simulink model "test_simu2"  (R2019a)
settings: Solver=VariableStepAuto  StartTime=0.0  StopTime=10.0  RelTol=1e-3
values from neighbouring files (symbols this model uses):
  b = 3.0 *10^-5    (= 3e-05)    [constants_drone.m]    (also in drone.m)
  d = 1.1*10^-6    (= 1.1e-06)    [constants_drone.m]    (also in drone.m)
  omega1 = 475    [constants_drone.m]
  omega2 = 500    [constants_drone.m]
  omega3 = 475    [constants_drone.m]
  omega4 = 475    [constants_drone.m]
undefined symbols (not defined in the file or in its folder): magnitude
settings Model: Creator=Emil  LastModifiedBy=Emil

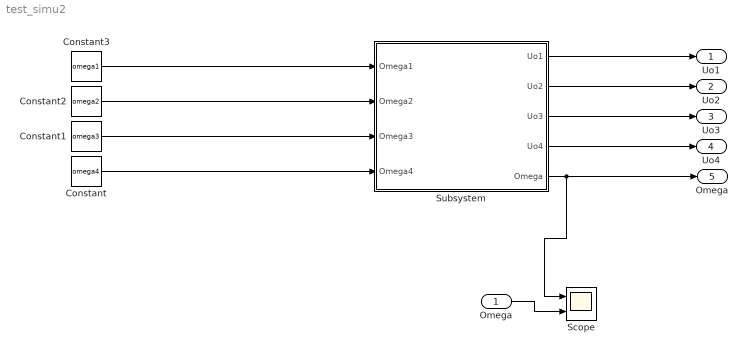
== system test_simu2 ==
  "Omega " : Inport
  Constant : Constant  Value=omega4
  Constant1 : Constant  Value=omega3
  Constant2 : Constant  Value=omega2
  Constant3 : Constant  Value=omega1
  Scope : Scope  NumInputPorts=2
  Subsystem : Subsystem
  Uo1 : Outport
  Uo2 : Outport  Port=2
  Uo3 : Outport  Port=3
  Uo4 : Outport  Port=4
  Omega : Outport  Port=5
  wires:
  Constant3/1 -> Subsystem/1(Omega1)
  Constant2/1 -> Subsystem/2(Omega2)
  Constant1/1 -> Subsystem/3(Omega3)
  Constant/1 -> Subsystem/4(Omega4)
  Subsystem/1(Uo1) -> Uo1/1
  Subsystem/2(Uo2) -> Uo2/1
  Subsystem/3(Uo3) -> Uo3/1
  Subsystem/4(Uo4) -> Uo4/1
  Subsystem/5(Omega) -> Scope/1, Omega/1
  "Omega "/1 -> Scope/2

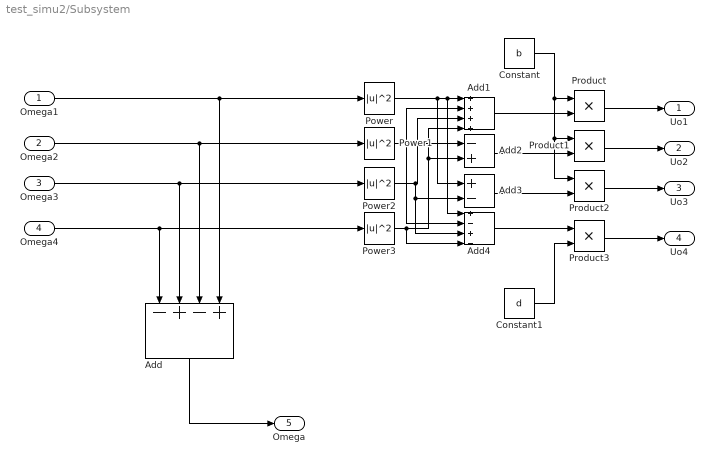
== system test_simu2/Subsystem ==
  Omega1 : Inport
  Omega2 : Inport  Port=2
  Omega3 : Inport  Port=3
  Omega4 : Inport  Port=4
  Add : Sum  Inputs=-+-+
  Add1 : Sum  Inputs=++++
  Add2 : Sum  Inputs=-+
  Add3 : Sum  Inputs=+-
  Add4 : Sum  Inputs=+-+-
  Constant : Constant  Value=b
  Constant1 : Constant  Value=d
  Power{,1..3} (4 alike) : Math  Operator=magnitude^2  SaturateOnIntegerOverflow=on
  Product{,1..3} (4 alike) : Product
  Uo1 : Outport
  Uo2 : Outport  Port=2
  Uo3 : Outport  Port=3
  Uo4 : Outport  Port=4
  Omega : Outport  Port=5
  wires:
  Add4/1 -> Product3/1
  Power3/1 -> Add4/4, Add2/2, Add1/4
  Omega4/1 -> Power3/1, Add/1
  Omega2/1 -> Add/3, Power1/1
  Omega1/1 -> Power/1, Add/4
  Power/1 -> Add3/1, Add4/1, Add1/1
  Omega3/1 -> Power2/1, Add/2
  Constant/1 -> Product2/1, Product1/1, Product/1
  Add2/1 -> Product1/2
  Constant1/1 -> Product3/2
  Product3/1 -> Uo4/1
  Product2/1 -> Uo3/1
  Power1/1 -> Add4/2, Add2/1, Add1/2
  Product1/1 -> Uo2/1
  Add3/1 -> Product2/2
  Power2/1 -> Add4/3, Add3/2, Add1/3
  Add1/1 -> Product/2
  Add/1 -> Omega/1
  Product/1 -> Uo1/1
